simulink model "ASD_votlage_control"  (R2021a)
settings: Solver=FixedStepDiscrete  StartTime=0.0  StopTime=1  FixedStep=1e-5  RelTol=1e-3
model workspace (MAT data in the model file):
  amplitue = 2
  x = 90
libraries: spsIGBTLib x12, spsThreePhaseSeriesRLCBranchLib x4, spsGroundLib x3, spsSeriesRLCBranchLib x2, spsThreePhaseVIMeasurementLib x2, spsMultimeterLib x1, simulink x1, spsThreePhaseParallelRLCBranchLib x1, spsThreePhaseSourceLib x1, spsVoltageMeasurementLib x1, spspowerguiLib x1
settings Model: Creator=Mehra  LastModifiedBy=Mehra
settings DebuggingCC: UnconnectedInputMsg=none  UnconnectedOutputMsg=none  UnconnectedLineMsg=none

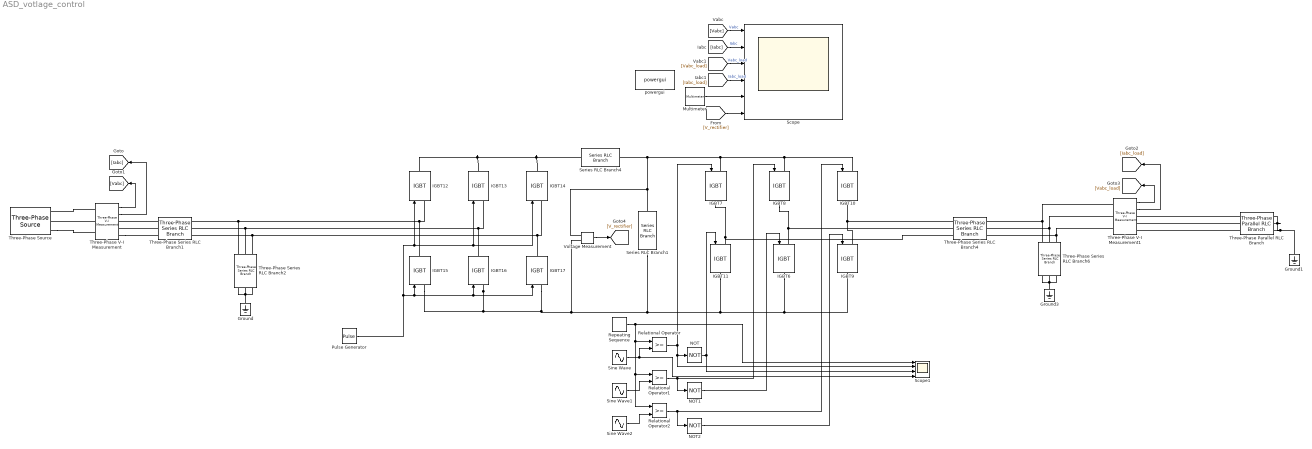
== system ASD_votlage_control ==
  Ground : spsGroundLib/Ground  LConnTagsString=a
  Ground1 : spsGroundLib/Ground  LConnTagsString=a
  Ground3 : spsGroundLib/Ground  LConnTagsString=a
  IGBT{6..17} (12 alike) : spsIGBTLib/IGBT  Ron=0.001  Lon=0  Vf=1  Tf=1e-6  Tt=2e-6  IC=0  Rs=1e5  Cs=inf  Measurements=off
  Multimeter : spsMultimeterLib/Multimeter  PhasorSimulation=off  OutputType=Complex  sel=2  L=2  Gain=1  yselected={'Ib: Series RLC Branch4'};  PSBOutputType=1  PSBequivalent=0  AxesSetting=[0,0.1,-100,100]  Display=0  SavedBlockNames=-11
  NOT : Logic  Operator=NOT  IconShape=distinctive  AllPortsSameDT=off  OutDataTypeStr=boolean
  NOT1 : Logic  Operator=NOT  IconShape=distinctive  AllPortsSameDT=off  OutDataTypeStr=boolean
  NOT2 : Logic  Operator=NOT  IconShape=distinctive  AllPortsSameDT=off  OutDataTypeStr=boolean
  Pulse Generator : DiscretePulseGenerator  PulseType=Time based  Period=0.01  PulseWidth=99
  Relational Operator : RelationalOperator  OutDataTypeStr=boolean  RndMeth=Simplest
  Relational Operator1 : RelationalOperator  OutDataTypeStr=boolean  RndMeth=Simplest
  Relational Operator2 : RelationalOperator  OutDataTypeStr=boolean  RndMeth=Simplest
  Repeating Sequence : simulink/Sources/Repeating Sequence  rep_seq_t=[0 1/5000]  rep_seq_y=[0 1]
  Scope : Scope  NumInputPorts=6
  Scope1 : Scope  NumInputPorts=4
  Series RLC Branch1 : spsSeriesRLCBranchLib/Series RLC Branch  LConnTagsString=__new0  RConnTagsString=__new0  BranchType=C  Resistance=10  Inductance=220e-6  SetiL0=off  InitialCurrent=0  Capacitance=220e-6  Setx0=off  InitialVoltage=0  Measurements=Branch current
  Series RLC Branch4 : spsSeriesRLCBranchLib/Series RLC Branch  LConnTagsString=__new0  RConnTagsString=__new0  BranchType=L  Resistance=10  Inductance=18e-6  SetiL0=off  InitialCurrent=0  Capacitance=4.7e-6  Setx0=off  InitialVoltage=0  Measurements=Branch current
  Sine Wave : Sin  Amplitude=amplitue  Frequency=2*pi*50  SampleTime=1e-5
  Sine Wave1 : Sin  Amplitude=amplitue  Frequency=2*pi*50  Phase=2*pi/3  SampleTime=1e-5
  Sine Wave2 : Sin  Amplitude=amplitue  Frequency=2*pi*50  Phase=4*pi/3  SampleTime=1e-5
  Three-Phase Parallel RLC Branch : spsThreePhaseParallelRLCBranchLib/Three-Phase Parallel RLC Branch  LConnTagsString=A|B|C  RConnTagsString=A|B|C  BranchType=RL  Resistance=5.4  Inductance=0.365  Capacitance=1e-6  Measurements=None
      settings: SourceProductBaseCode=PS
  Three-Phase Series RLC Branch1 : spsThreePhaseSeriesRLCBranchLib/Three-Phase Series RLC Branch  LConnTagsString=A|B|C  RConnTagsString=A|B|C  BranchType=L  Resistance=1  Inductance=470e-6  Capacitance=470e-6  Measurements=None
  Three-Phase Series RLC Branch2 : spsThreePhaseSeriesRLCBranchLib/Three-Phase Series RLC Branch  LConnTagsString=A|B|C  RConnTagsString=A|B|C  BranchType=C  Resistance=1  Inductance=1e-3  Capacitance=100e-6  Measurements=None
  Three-Phase Series RLC Branch4 : spsThreePhaseSeriesRLCBranchLib/Three-Phase Series RLC Branch  LConnTagsString=A|B|C  RConnTagsString=A|B|C  BranchType=L  Resistance=1  Inductance=74e-6  Capacitance=470e-6  Measurements=None
  Three-Phase Series RLC Branch6 : spsThreePhaseSeriesRLCBranchLib/Three-Phase Series RLC Branch  LConnTagsString=A|B|C  RConnTagsString=A|B|C  BranchType=C  Resistance=1  Inductance=1e-3  Capacitance=100e-6  Measurements=None
  Three-Phase V-I Measurement : spsThreePhaseVIMeasurementLib/Three-Phase V-I Measurement  VoltageMeasurement=phase-to-ground  SetLabelV=off  LabelV=Vabc  Vpu=off  VpuLL=off  CurrentMeasurement=yes  SetLabelI=off  LabelI=Iabc  Ipu=off  Pbase=100e6  Vbase=500e3  OutputType=Complex  PhasorSimulation=off  PSBequivalent=0
  Three-Phase V-I Measurement1 : spsThreePhaseVIMeasurementLib/Three-Phase V-I Measurement  VoltageMeasurement=phase-to-ground  SetLabelV=off  LabelV=Vabc  Vpu=off  VpuLL=off  CurrentMeasurement=yes  SetLabelI=off  LabelI=Iabc  Ipu=off  Pbase=100e6  Vbase=500e3  OutputType=Complex  PhasorSimulation=off  PSBequivalent=0
  Three-Phase Source : spsThreePhaseSourceLib/Three-Phase Source  InternalConnection=Yg  VoltagePhases=off  Voltage=400  PhaseAngle=0  Voltage_phases=[25e3 25e3 25e3]/sqrt(3)  PhaseAngles_phases=[0 -120 +120]  Frequency=50  NonIdealSource=on  SpecifyImpedance=off  Resistance=0.89e-3  Inductance=16.58e-6  ShortCircuitLevel=100e6  BaseVoltage=415  XRratio=7  BusType=swing  Pref=10e3  Qref=0  Prefabc=[10e3, 10e3, 10e3]  Qrefabc=[0, 0, 0]  Qmin=-inf  Qmax=inf
  Voltage Measurement : spsVoltageMeasurementLib/Voltage Measurement  PhasorSimulation=off  OutputType=Complex  PSBequivalent=0
  powergui : spspowerguiLib/powergui  Priority=1  SimulationMode=Discrete  SampleTime=1e-5  frequency=60  Iterations=50  frequencyindice=0  Pbase=100e6  ErrMax=1e-4  UnitsV=kV  UnitsW=MW  buscounter=0  FunctionMessages=off  echomessages=off  EnableUseOfTLC=off  CurrentSourceSwitches=off  DisableSnubberDevices=off  DisableRonSwitches=off  DisableVfSwitches=off  DisplayEquations=off  AutomaticDiscreteSolvers=off  SolverType=Tustin/Backward Euler (TBE)  Interpol=off  ExternalGateDelay=off  methode=off  Ts=100  x0status=blocks  SPID=on  SwTol=0  HookPort=off  NonlinearTolerance=1e-4  nMaxIteration=100  ContinueOnMaxIteration=off  RestoreLinks=warning  ResistiveCurrentMeasurement=off  Frange=[0:2:500]  Ylog=off  Xlog=on  ShowGrid=off  save=off  variable=ZData  structure=0  ZoomFFT=off  StartTime=0.0  cycles=1  DisplayStyle=1  fundamental=60  FreqAxis=off  MaxFrequency=1000  frequencyindicesteady=1  RmsSteady=1  display=off
  wires:
  [Vabc] -> Scope/1  "Vabc"
  [Iabc] -> Scope/2  "Iabc"
  Repeating Sequence/1 -> Relational Operator2/1, Relational Operator1/1, Relational Operator/1, Scope1/1
  Sine Wave/1 -> Scope1/4, Relational Operator/2
  Sine Wave1/1 -> Relational Operator1/2
  Sine Wave2/1 -> Relational Operator2/2
  Relational Operator/1 -> Scope1/2, NOT/1, IGBT7/1
  Relational Operator1/1 -> IGBT8/1, NOT1/1
  Relational Operator2/1 -> IGBT10/1, NOT2/1
  NOT/1 -> Scope1/3, IGBT11/1
  NOT1/1 -> IGBT6/1
  NOT2/1 -> IGBT9/1
  Three-Phase V-I Measurement1/2 -> [Iabc_load]
  Three-Phase V-I Measurement1/1 -> [Vabc_load]
  [Vabc_load] -> Scope/3  "Vabc_load"
  [Iabc_load] -> Scope/4  "Iabc_load"
  Multimeter/1 -> Scope/5
  Voltage Measurement/1 -> [V_rectifier]
  [V_rectifier] -> Scope/6
  Three-Phase V-I Measurement/2 -> [Iabc]
  Three-Phase V-I Measurement/1 -> [Vabc]
  Pulse Generator/1 -> IGBT14/1, IGBT13/1, IGBT12/1, IGBT17/1, IGBT16/1, IGBT15/1
  connections:
  IGBT7/LConn1 -- Voltage Measurement/LConn1 -- Series RLC Branch1/LConn1 -- Series RLC Branch4/RConn1 -- IGBT8/LConn1 -- IGBT10/LConn1
  Three-Phase Parallel RLC Branch/LConn1 -- Three-Phase V-I Measurement1/RConn1
  Three-Phase Parallel RLC Branch/LConn2 -- Three-Phase V-I Measurement1/RConn2
  Three-Phase Parallel RLC Branch/LConn3 -- Three-Phase V-I Measurement1/RConn3
  Ground1/LConn1 -- Three-Phase Parallel RLC Branch/RConn1 -- Three-Phase Parallel RLC Branch/RConn2 -- Three-Phase Parallel RLC Branch/RConn3
  IGBT17/LConn1 -- IGBT6/RConn1 -- IGBT9/RConn1 -- IGBT11/RConn1 -- Series RLC Branch1/RConn1 -- Voltage Measurement/LConn2 -- IGBT15/LConn1 -- IGBT16/LConn1
  IGBT9/LConn1 -- IGBT10/RConn1 -- Three-Phase Series RLC Branch4/LConn1
  IGBT7/RConn1 -- Three-Phase Series RLC Branch4/LConn3 -- IGBT11/LConn1
  Three-Phase Series RLC Branch6/RConn2 -- Three-Phase Series RLC Branch6/RConn3 -- Ground3/LConn1 -- Three-Phase Series RLC Branch6/RConn1
  Three-Phase Series RLC Branch6/LConn2 -- Three-Phase V-I Measurement1/LConn2 -- Three-Phase Series RLC Branch4/RConn2
  IGBT8/RConn1 -- Three-Phase Series RLC Branch4/LConn2 -- IGBT6/LConn1
  Three-Phase Series RLC Branch6/LConn1 -- Three-Phase V-I Measurement1/LConn1 -- Three-Phase Series RLC Branch4/RConn1
  Three-Phase Series RLC Branch6/LConn3 -- Three-Phase V-I Measurement1/LConn3 -- Three-Phase Series RLC Branch4/RConn3
  IGBT14/RConn1 -- Series RLC Branch4/LConn1 -- IGBT13/RConn1 -- IGBT12/RConn1
  Three-Phase Series RLC Branch2/RConn3 -- Three-Phase Series RLC Branch2/RConn1 -- Ground/LConn1 -- Three-Phase Series RLC Branch2/RConn2
  Three-Phase Series RLC Branch1/RConn3 -- Three-Phase Series RLC Branch2/LConn3 -- IGBT14/LConn1 -- IGBT17/RConn1
  Three-Phase Series RLC Branch1/RConn2 -- Three-Phase Series RLC Branch2/LConn2 -- IGBT13/LConn1 -- IGBT16/RConn1
  Three-Phase Series RLC Branch2/LConn1 -- Three-Phase Series RLC Branch1/RConn1 -- IGBT15/RConn1 -- IGBT12/LConn1
  Three-Phase V-I Measurement/LConn2 -- Three-Phase Source/RConn2
  Three-Phase Series RLC Branch1/LConn2 -- Three-Phase V-I Measurement/RConn2
  Three-Phase V-I Measurement/RConn3 -- Three-Phase Series RLC Branch1/LConn3
  Three-Phase V-I Measurement/LConn1 -- Three-Phase Source/RConn1
  Three-Phase Series RLC Branch1/LConn1 -- Three-Phase V-I Measurement/RConn1
  Three-Phase Source/RConn3 -- Three-Phase V-I Measurement/LConn3
